simulink model "Design_model_MOD"  (R2025b)
settings: Solver=FixedStepAuto  StartTime=0.0  StopTime=Tf  FixedStep=Ts  RelTol=1e-3
values from neighbouring files (symbols this model uses):
  Ki = (Time_const/Km)*W_cl^2    (= 54.4581574453)    [Stabilization_MOD.m]
  Km = 12.4132 / 12.7177    (= 0.976056991437)    [Stabilization_MOD.m]
  Kp = (2*W_cl*Zeta_cl*Time_const - 1)/Km    [Stabilization_MOD.m]
  Sim_disturbance_amplitude = 8    [Stabilization_MOD.m]
  Sim_disturbance_freq = pi    (= 3.14159265359)    [Stabilization_MOD.m]
  Time_const = 1 / 12.7177    (= 0.078630569993)    [Stabilization_MOD.m]
  Tsample = 0.005    [Stabilization_MOD.m]
settings Model: Creator=GILBERT  LastModifiedBy=GILBERT

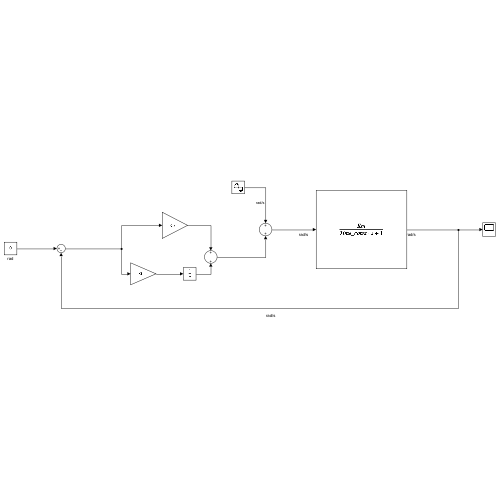
[thumbnail: Simulink's stored preview of the top-level diagram]
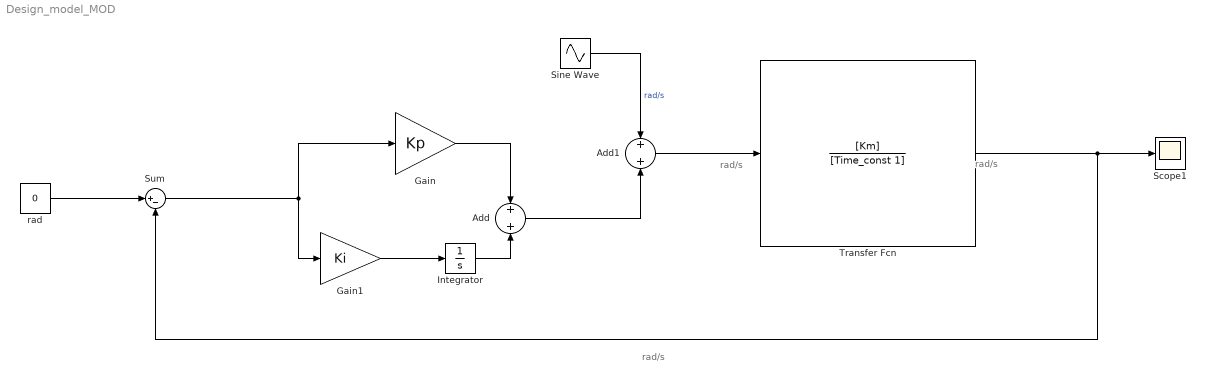
== system Design_model_MOD ==
  note: rad/s
  note: rad/s
  note: rad/s
  Add : Sum
  Add1 : Sum
  Gain : Gain  Gain=Kp
  Gain1 : Gain  Gain=Ki
  Integrator : Integrator
  Scope1 : Scope
      settings: ActiveDisplayYMinimum=-1.0331029561247216  ActiveDisplayYMaximum=1.0161945669030548
  Sine Wave : Sin  Amplitude=Sim_disturbance_amplitude  Frequency=Sim_disturbance_freq  SampleTime=Tsample
  Sum : Sum  Inputs=|+-
  Transfer Fcn : TransferFcn  Numerator=[Km]  Denominator=[Time_const 1]
  rad : Constant  Value=0
  wires:
  Gain/1 -> Add/1
  Gain1/1 -> Integrator/1
  Integrator/1 -> Add/2
  Sum/1 -> Gain1/1, Gain/1
  rad/1 -> Sum/1
  Add/1 -> Add1/2
  Add1/1 -> Transfer Fcn/1
  Sine Wave/1 -> Add1/1  "rad/s"
  Transfer Fcn/1 -> Sum/2, Scope1/1
